simulink model "DistillationColumn"  (R2024a)
settings: Solver=ode23s  StartTime=0.0  StopTime=tfinal  RelTol=1e-3
undefined symbols (not defined in the file): L, V
settings Model: Creator=tmlouw  LastModifiedBy=tmlouw

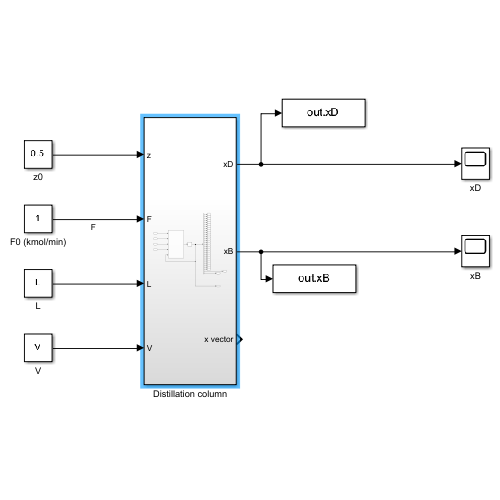
[thumbnail: Simulink's stored preview of the top-level diagram]
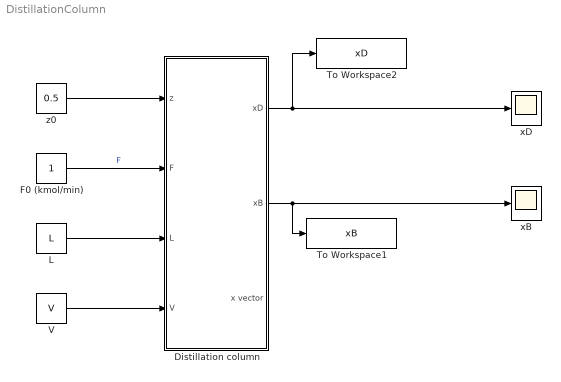
== system DistillationColumn ==
  Distillation column : Subsystem
  F0 (kmol/min) : Constant
  L : Constant  Value=L
  To Workspace1 : ToWorkspace  VariableName=xB  SampleTime=10
      settings: Save2DSignal=2-D array (concatenate along first dimension)
  To Workspace2 : ToWorkspace  VariableName=xD  SampleTime=10
      settings: Save2DSignal=2-D array (concatenate along first dimension)
  V : Constant  Value=V
  xB : Scope
  xD : Scope
  z0 : Constant  Value=0.5
  wires:
  z0/1 -> Distillation column/1(z)
  F0 (kmol/min)/1 -> Distillation column/2(F)  "F"
  Distillation column/1(xD) -> xD/1, To Workspace2/1
  Distillation column/2(xB) -> To Workspace1/1, xB/1
  V/1 -> Distillation column/4(V)
  L/1 -> Distillation column/3(L)

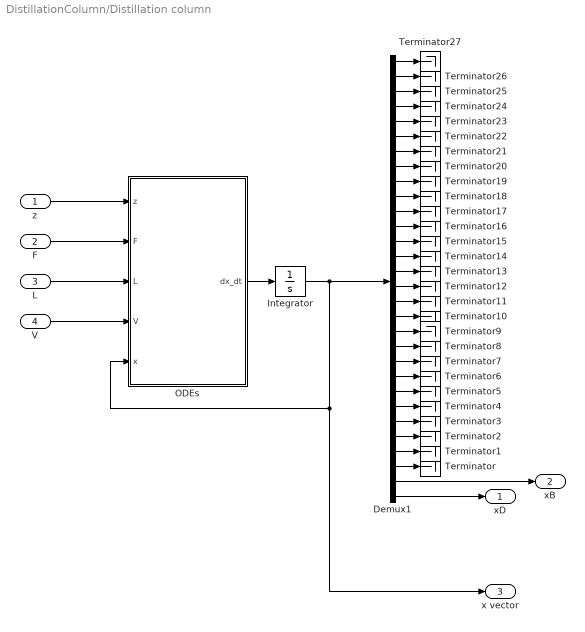
== system DistillationColumn/Distillation column ==
  z : Inport
  F : Inport  Port=2
  L : Inport  Port=3
  V : Inport  Port=4
  Demux1 : Demux  Outputs=30
  Integrator : Integrator  InitialCondition=[linspace(0,0.99,28)'; 0.036; 0.96]  UpperSaturationLimit=1  LowerSaturationLimit=0
  ODEs : MATLAB Function  TreatAsAtomicUnit=on
  Terminator{,1..27} (28 alike) : Terminator
  xD : Outport
  xB : Outport  Port=2
  x vector : Outport  Port=3
  wires:
  F/1 -> ODEs/2(F)
  V/1 -> ODEs/4(V)
  ODEs/1(dx_dt) -> Integrator/1
  Demux1/29 -> xB/1
  L/1 -> ODEs/3(L)
  Demux1/30 -> xD/1
  z/1 -> ODEs/1(z)
  Demux1/20 -> Terminator8/1
  Demux1/16 -> Terminator12/1
  Demux1/14 -> Terminator14/1
  Demux1/17 -> Terminator11/1
  Demux1/23 -> Terminator5/1
  Demux1/9 -> Terminator19/1
  Demux1/8 -> Terminator20/1
  Demux1/11 -> Terminator17/1
  Demux1/12 -> Terminator16/1
  Demux1/27 -> Terminator1/1
  Demux1/1 -> Terminator27/1
  Demux1/13 -> Terminator15/1
  Demux1/6 -> Terminator22/1
  Integrator/1 -> x vector/1, ODEs/5(x), Demux1/1
  Demux1/4 -> Terminator24/1
  Demux1/19 -> Terminator9/1
  Demux1/24 -> Terminator4/1
  Demux1/25 -> Terminator3/1
  Demux1/5 -> Terminator23/1
  Demux1/18 -> Terminator10/1
  Demux1/2 -> Terminator26/1
  Demux1/28 -> Terminator/1
  Demux1/10 -> Terminator18/1
  Demux1/7 -> Terminator21/1
  Demux1/26 -> Terminator2/1
  Demux1/21 -> Terminator7/1
  Demux1/15 -> Terminator13/1
  Demux1/22 -> Terminator6/1
  Demux1/3 -> Terminator25/1

== matlab function DistillationColumn/Distillation column/ODEs ==
  data: z input; dx_dt output; F input; L input; V input; x input
function dx_dt = distillationColumn(z, F, L, V, x)
% ODEs representing a 30-tray distillation column for benzene/toluene
% separation. All molar hold-ups are constant, only composition varies.
% The feed is assumed to be a saturated liquid.
%
% Inputs are defined as follows:
%   z: ~, feed composition
%   F: kmol/min, feed flowrate
%   L: kmol/min, reflux flowrate
%   V: kmol/min, vapour flowrate
% Input "x" has 30 elements
%   x(1:28): ~, composition on stages 1-28
%   x(29): ~, bottoms composition
%   x(30): ~, condenser composition

nB = 100;  % kmol, molar hold-up in reboiler
n = 10;    % kmol, molar hold-up per tray
nD = 100;  % kmol, molar hold-up in condenser

N = 28; % ~, Number of stages
f = 15; % ~, Feed stage

xB = x(29); % ~, bottoms composition
xD = x(30); % ~, distillate composition
LB = L + F;    % kmol/min, liquid flowrate below feed tray
B = L + F - V; % kmol/min, bottoms flowrate

alpha = 2.5; % ~, relative volatility
fy = @(x) alpha*x / (1 + (alpha-1)*x); % ~, vapour composition given specified liquid composition "x"

% Calculate the vapour composition on each tray, as well as over the reboiler
y = zeros(28,1);
for i = 1:N
    y(i) = fy(x(i));
end
yB = fy(xB);

% Create an empty array representing the derivative of composition wrt time
dx_dt = zeros(30,1);

% Calculate time rate of change of composition for the reboiler, each tray,
% and the distillate, using a molar balance over each
% Reboiler and first stage
dxB_dt = ( LB*x(1) - B*xB - V*yB )/nB;
dx_dt(1) = ( LB*(x(2) - x(1)) + V*(yB - y(1)) )/n;
% Below feed
for i = 2:f-1
    dx_dt(i) = ( LB*(x(i+1) - x(i)) + V*(y(i-1) - y(i)) )/n;
end
% Feed stage
dx_dt(f) = ( F*z + L*x(f+1) - LB*x(f) + V*(y(f-1) - y(f)) )/n;
% Above feed
for i = f+1:N-1
    dx_dt(i) = ( L*(x(i+1) - x(i)) + V*(y(i-1) - y(i)) )/n;
end
% Top stage and condenser
dx_dt(N) =  ( L*(xD - x(N)) + V*(y(N-1) - y(N)) )/n;
dxD_dt = V*(y(N) - xD)/nD;

dx_dt(29) = dxB_dt;
dx_dt(30) = dxD_dt;
